simulink model "GFLIB_ControllerPIr_BAM"  (Simulink 9.3)
settings: Solver=VariableStepAuto  StartTime=0.0  StopTime=10.0  RelTol=1e-3
settings Model: Creator=nxa18952  LastModifiedBy=nxa18952
settings DataIOCC: SaveFormat=Dataset  SignalLoggingSaveFormat=Dataset  ReturnWorkspaceOutputs=on
settings OptimizationCC: LifeSpan=auto
settings DebuggingCC: UnderspecifiedInitializationDetection=Simplified  MergeDetectMultiDrivingBlocksExec=error  FcnCallInpInsideContextMsg=error  SFUnexpectedBacktrackingDiag=error  SFNoUnconditionalDefaultTransitionDiag=error  SFExecutionAtInitializationDiag=warning  ArithmeticOperatorsInVariantConditions=error
settings HardwareCC: ProdBitPerPointer=64  ProdBitPerSizeT=64  ProdBitPerPtrDiffT=64  ProdLargestAtomicFloat=Float  ProdIntDivRoundTo=Zero  ProdEndianess=LittleEndian  ProdWordSize=64  ProdHWDeviceType=Intel->x86-64 (Windows64)
settings ModelReferenceCC: PropagateSignalLabelsOutOfModel=on
settings SFSimCC: SimUseLocalCustomCode=on
settings RTWCC: RTWUseLocalCustomCode=on
settings CodeAppCC: StateflowObjectComments=off
settings GRTTargetCC: TargetLangStandard=C99 (ISO)  CombineOutputUpdateFcns=on  GRTInterface=off
settings ConfigComp: CovMetricSettings=dwe  CovHtmlReporting=off  CovSaveCumulativeToWorkspaceVar=off  CovSaveSingleToWorkspaceVar=off  CovExternalEMLEnable=on

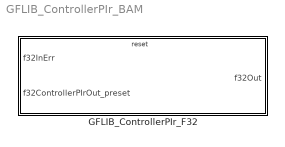
== system GFLIB_ControllerPIr_BAM ==
  GFLIB_ControllerPIr_F32 : Subsystem  TreatAsAtomicUnit=on  mask(GFLIB_ControllerPIr_F32){showStates=Hide (faster execution), resetStatesEnable=Pre-set according to the first set of inputs after reset, f32CC1=0, f32CC2=0, u16NShift=0}
      mask prompts: showStates "Show internal states"; resetStatesEnable "Internal state after reset"; f32CC1 "f32CC1 (CC1 coefficient)"; f32CC2 "f32CC2 (CC2 coefficient)"; u16NShift "u16NShift (Scaling bitwise shift applied to the controller coefficients)"
      mask help: Reccurent form PI controller without anti-windup in 32-bit fixed-point fractional implementation. This block supports re-initialization of the internal state during simulation. If the block is reset, the controller's output will be aligned with the input f32ControllerPIrOut_preset. Refer to the AMMCLIB User's Guide for further details.
      mask init:
      | if ~evalin('base','exist(''tS8'',''var'')')
      |   if (2 ~= exist('SWLIBS_Typedefs.mat','file'))
      |       error('File SWLIBS_Typedefs.mat is not on the Matlab path. Please add the AMMCLIB "bam" folder in the Matlab Search Path.');
      |   else
      |       evalin('base', 'load(''SWLIBS_Typedefs.mat'')');
      |   end
      | end
      | if showStates == 1
      |     % hidden state variables
      |     if strcmp(get_param([gcb '/f32CC1sc'], 'BlockType'), 'Inport')
      |         posblk = get_param(gcb, 'Position');
      | 
      |         pos = get_param(    [gcb, '/f32CC1sc'], 'Position');
      |         orient = get_param( [gcb, '/f32CC1sc'], 'Orientation');
      |         delete_block(       [gcb, '/f32CC1sc']);
      |         add_block('built-in/Ground', [gcb, '/f32CC1sc'], 'Position', pos, 'Orientation', orient);
      | 
      |         pos = get_param(    [gcb, '/f32CC2sc'], 'Position');
      |         orient = get_param( [gcb, '/f32CC2sc'], 'Orientation');
      |         delete_block(       [gcb, '/f32CC2sc']);
      |         add_block('built-in/Ground', [gcb, '/f32CC2sc'], 'Position', pos, 'Orientation', orient);
      | 
      |         pos = get_param(    [gcb, '/f32Acc'], 'Position');
      |         orient = get_param( [gcb, '/f32Acc'], 'Orientation');
      |         delete_block(       [gcb, '/f32Acc']);
      |         add_block('built-in/Ground', [gcb, '/f32Acc'], 'Position', pos, 'Orientation', orient);
      | 
      |         pos = get_param(    [gcb, '/f32InErrK1'], 'Position');
      |         orient = get_param( [gcb, '/f32InErrK1'], 'Orientation');
      |         delete_block(       [gcb, '/f32InErrK1']);
      |         add_block('built-in/Ground', [gcb, '/f32InErrK1'], 'Position', pos, 'Orientation', orient);
      | 
      |         pos = get_param(    [gcb, '/u16NShift'], 'Position');
      |         orient = get_param( [gcb, '/u16NShift'], 'Orientation');
      |         delete_block(       [gcb, '/u16NShift']);
      |         add_block('built-in/Ground', [gcb, '/u16NShift'], 'Position', pos, 'Orientation', orient);
      | 
      | 
      |         pos = get_param(    [gcb '/f32Acc_Out'], 'Position');
      |         orient = get_param( [gcb '/f32Acc_Out'], 'Orientation');
      |         delete_block(       [gcb '/f32Acc_Out']);
      |         add_block('built-in/Terminator', [gcb '/f32Acc_Out'], 'Position', pos, 'Orientation', orient);
      | 
      |         pos = get_param(    [gcb '/f32InErrK1_Out'], 'Position');
      |         orient = get_param( [gcb '/f32InErrK1_Out'], 'Orientation');
      |         delete_block(       [gcb '/f32InErrK1_Out']);
      |         add_block('built-in/Terminator', [gcb '/f32InErrK1_Out'], 'Position', pos, 'Orientation', orient);
      | 
      | 
      |         set_param([gcb '/f32InErr'], 'Port', '1');
      |         set_param([gcb '/f32ControllerPIrOut_preset'], 'Port', '2');
      | 
      |         set_param([gcb '/f32Out'], 'Port', '1');
      | 
      |         set_param(gcb,'MaskEnables',{'on','on','on','on','on'});
      | 
      |         if (posblk(4) - posblk(2)) > 75
      |           height = 75;
      |           set_param(gcb,'Position',[posblk(1), posblk(2), posblk(3), posblk(2)+height])
      |         end
      |     end
      | else
      |     % shown state variables
      |     if strcmp(get_param([gcb '/f32CC1sc'], 'BlockType'), 'Ground')
      |         posblk = get_param(gcb, 'Position');
      | 
      |         pos = get_param(    [gcb, '/f32CC1sc'], 'Position');
      |         orient = get_param( [gcb, '/f32CC1sc'], 'Orientation');
      |         delete_block(       [gcb, '/f32CC1sc']);
      |         add_block('built-in/Inport', [gcb, '/f32CC1sc'], 'Position', pos, 'Orientation', orient, 'OutDataTypeStr', 'int32');
      | 
      |         pos = get_param(    [gcb, '/f32CC2sc'], 'Position');
      |         orient = get_param( [gcb, '/f32CC2sc'], 'Orientation');
      |         delete_block(       [gcb, '/f32CC2sc']);
      |         add_block('built-in/Inport', [gcb, '/f32CC2sc'], 'Position', pos, 'Orientation', orient, 'OutDataTypeStr', 'int32');
      | 
      |         pos = get_param(    [gcb, '/f32Acc'], 'Position');
      |         orient = get_param( [gcb, '/f32Acc'], 'Orientation');
      |         delete_block(       [gcb, '/f32Acc']);
      |         add_block('built-in/Inport', [gcb, '/f32Acc'], 'Position', pos, 'Orientation', orient, 'OutDataTypeStr', 'int32');
      | 
      |         pos = get_param(    [gcb, '/f32InErrK1'], 'Position');
      |         orient = get_param( [gcb, '/f32InErrK1'], 'Orientation');
      |         delete_block(       [gcb, '/f32InErrK1']);
      |         add_block('built-in/Inport', [gcb, '/f32InErrK1'], 'Position', pos, 'Orientation', orient, 'OutDataTypeStr', 'int32');
      | 
      |         pos = get_param(    [gcb, '/u16NShift'], 'Position');
      |         orient = get_param( [gcb, '/u16NShift'], 'Orientation');
      |         delete_block(       [gcb, '/u16NShift']);
      |         add_block('built-in/Inport', [gcb, '/u16NShift'], 'Position', pos, 'Orientation', orient, 'OutDataTypeStr', 'uint16');
      | 
      | 
      |         pos = get_param(    [gcb '/f32Acc_Out'], 'Position');
      |         orient = get_param( [gcb '/f32Acc_Out'], 'Orientation');
      |         delete_block(       [gcb '/f32Acc_Out']);
      |         add_block('built-in/Outport', [gcb '/f32Acc_Out'], 'Position', pos, 'Orientation', orient);
      | 
      |         pos = get_param(    [gcb '/f32InErrK1_Out'], 'Position');
      |         orient = get_param( [gcb '/f32InErrK1_Out'], 'Orientation');
      |         delete_block(       [gcb '/f32InErrK1_Out']);
      |         add_block('built-in/Outport', [gcb '/f32InErrK1_Out'], 'Position', pos, 'Orientation', orient);
      | 
      | 
      |         set_param([gcb '/f32InErr'], 'Port', '1');
      |         set_param([gcb '/f32ControllerPIrOut_preset'], 'Port', '2');
      |         set_param([gcb '/f32CC1sc'], 'Port', '3');
      |         set_param([gcb '/f32CC2sc'], 'Port', '4');
      |         set_param([gcb '/f32Acc'], 'Port', '5');
      |         set_param([gcb '/f32InErrK1'], 'Port', '6');
      |         set_param([gcb '/u16NShift'], 'Port', '7');
      | 
      |         set_param([gcb '/f32Out'], 'Port', '1');
      |         set_param([gcb '/f32Acc_Out'], 'Port', '2');
      |         set_param([gcb '/f32InErrK1_Out'], 'Port', '3');
      | 
      |         set_param(gcb,'MaskEnables',{'on','on','off','off','off'});
      | 
      |         if (posblk(4) - posblk(2)) < 200
      |           height = 200;
      |           set_param(gcb,'Position',[posblk(1), posblk(2), posblk(3), posblk(2)+height])
      |         end
      |     end
      | end
      settings: RTWSystemCode=Inline
      mask TypeOptions showStates: Hide (faster execution) | Show (allows debugging; connect feedback loops manually)
      mask Callback showStates:
      | maskStr = get_param(gcb,'showStates');
      | if strcmp(maskStr,'Hide (faster execution)'),
      |     set_param(gcb,'MaskEnables',{'on','on','on','on','on'});
      | else
      |     set_param(gcb,'MaskEnables',{'on','on','off','off','off'});
      | end
      mask TypeOptions resetStatesEnable: Pre-set according to the first set of inputs after reset | Clear to zero
      mask Display:
      | color('black');
      | pos = get_param(gcb, 'Position');
      | width = pos(3) - pos(1);
      | height = pos(4) - pos(2);
      | tX=width/2;
      | tY=height - 25;
      | color('black');
      | text(tX,tY, 'GFLIB_ControllerPIr_F32', 'horizontalAlignment', 'center');
      | if showStates == 2
      |   color('red');
      |   text(tX,tY - 20, ['debugging mode' char(13) char(10) '(limited performance)'], 'horizontalAlignment', 'center');
      | end

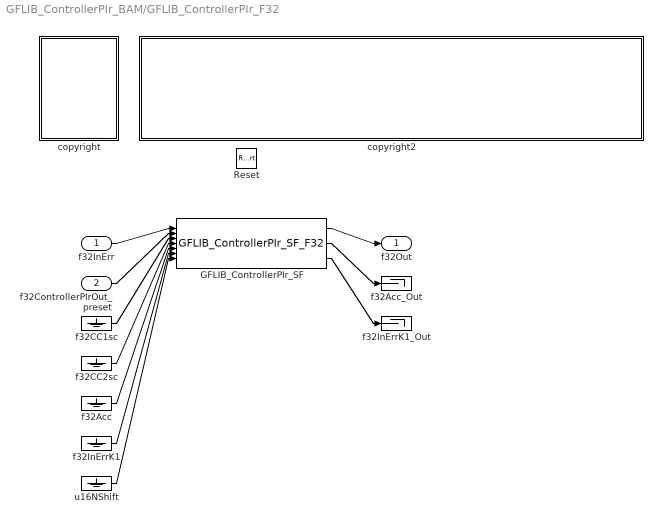
== system GFLIB_ControllerPIr_BAM/GFLIB_ControllerPIr_F32 ==
  f32InErr : Inport  OutDataTypeStr=int32
  f32ControllerPIrOut_preset : Inport  Port=2  OutDataTypeStr=int32
  Reset : ResetPort  DisableCoverage=on
  GFLIB_ControllerPIr_SF : S-Function  FunctionName=GFLIB_ControllerPIr_SF_F32  Parameters=showStates,resetStatesEnable,f32CC1,f32CC2,u16NShift  SFunctionDeploymentMode=off  EnableBusSupport=off
  copyright : Subsystem
      mask Display: text(10,90,'FILE:');text(10,75,'DESRIPTION:');text(10,60,'COPYRIGHT:');text(10,45,'VERSION:');text(10,30,'DATE:')
  copyright2 : Subsystem
      mask Display: text(10,90,'GFLIB_ControllerPIr_BAM_F32.mdl');text(10,75,'Recurrent form PI controller without anti-windup.');text(10,60,'NXP 2020');text(10,45,'1.0');text(10,30,'28-Mar-2020');
  f32Acc : Ground
  f32Acc_Out : Terminator
  f32CC1sc : Ground
  f32CC2sc : Ground
  f32InErrK1 : Ground
  f32InErrK1_Out : Terminator
  u16NShift : Ground
  f32Out : Outport
  wires:
  f32InErr/1 -> GFLIB_ControllerPIr_SF/1
  f32ControllerPIrOut_preset/1 -> GFLIB_ControllerPIr_SF/2
  f32CC1sc/1 -> GFLIB_ControllerPIr_SF/3
  f32CC2sc/1 -> GFLIB_ControllerPIr_SF/4
  f32Acc/1 -> GFLIB_ControllerPIr_SF/5
  f32InErrK1/1 -> GFLIB_ControllerPIr_SF/6
  u16NShift/1 -> GFLIB_ControllerPIr_SF/7
  GFLIB_ControllerPIr_SF/1 -> f32Out/1
  GFLIB_ControllerPIr_SF/2 -> f32Acc_Out/1
  GFLIB_ControllerPIr_SF/3 -> f32InErrK1_Out/1

== system GFLIB_ControllerPIr_BAM/GFLIB_ControllerPIr_F32/copyright ==

== system GFLIB_ControllerPIr_BAM/GFLIB_ControllerPIr_F32/copyright2 ==
